simulink model "cranesimu3"  (R2015a)
settings: Solver=ode45  StartTime=0.0  StopTime=25.0  RelTol=1e-3
InitFcn:
  | cranecontrol
undefined symbols (not defined in the file or in its folder): Grx, rrx
libraries: cstblocks x6
settings Model: Creator=roevhat  LastModifiedBy=roevhat

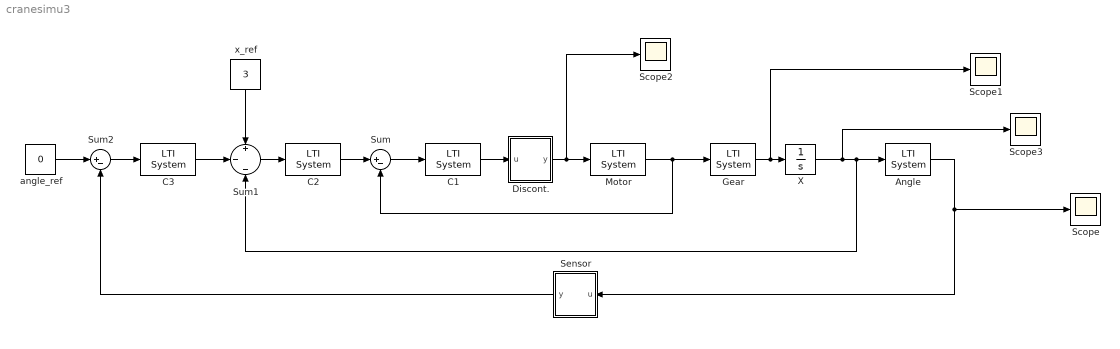
== system cranesimu3 ==
  Angle : cstblocks/LTI System  sys=W  IC=[]
  "C1 " : cstblocks/LTI System  sys=C1  IC=[]
  C2 : cstblocks/LTI System  sys=C2  IC=[]
  C3 : cstblocks/LTI System  sys=C3  IC=[]
  Discont. : MATLAB Function  TreatAsAtomicUnit=on
  Gear : cstblocks/LTI System  sys=Grx*rrx  IC=[]
  Motor : cstblocks/LTI System  sys=Mx  IC=[]
  Scope{,1..3} (4 alike) : Scope
      Scope settings: TimeRange=25  YMin=-0.25  YMax=-0.08
      Scope2 settings: SaveName=ScopeData2
      Scope3 settings: SaveName=ScopeData3
  Sensor : MATLAB Function  TreatAsAtomicUnit=on
  Sum : Sum  Inputs=|+-
  Sum1 : Sum  Inputs=+|-|-
  Sum2 : Sum  Inputs=|+-
  X : Integrator
  angle_ref : Constant  Value=0
  x_ref : Constant  Value=3
  wires:
  C2/1 -> Sum/1
  Sum/1 -> "C1 "/1
  Motor/1 -> Sum/2, Gear/1
  Gear/1 -> Scope1/1, X/1
  X/1 -> Scope3/1, Sum1/3, Angle/1
  Sum1/1 -> C2/1
  Sum2/1 -> C3/1
  Angle/1 -> Sensor/1(u), Scope/1
  angle_ref/1 -> Sum2/1
  x_ref/1 -> Sum1/1
  C3/1 -> Sum1/2
  "C1 "/1 -> Discont./1(u)
  Discont./1(y) -> Scope2/1, Motor/1
  Sensor/1(y) -> Sum2/2

== matlab function cranesimu3/Sensor ==
  data: u input; y output
function y = sensor(u)
    noise = 0.027 * (2*rand()-1);
    y = u + noise;
end

== matlab function cranesimu3/Discont. ==
  data: u input; y output
function y = dis(u)
    if(u > -4 && u < -0.5)
        y = -4;
    elseif(u < 4 && u > 0.5)
        y = 4;
    elseif(u > 12.5)
        y = 12.5;
    elseif(u < -12.5)
        y = -12.5;
    else
        y = u;
end
